simulink model "ProposedProblem1"  (R2013a)
settings: Solver=ode45  StartTime=0.0  StopTime=100  RelTol=1e-3
undefined symbols (not defined in the file): des, gcbh
settings Model: Creator=gabig  LastModifiedBy=gabig

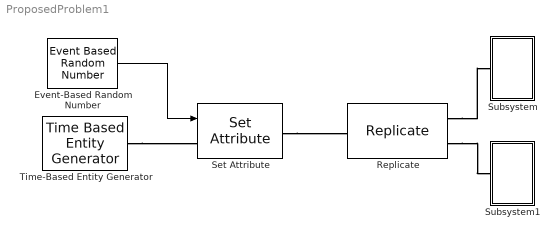
== system ProposedProblem1 ==
  Event-Based Random Number : EventBasedRandomNumber  Seed=14237
  Replicate : Replicate  NumberOutputPorts=2
  Set Attribute : SetAttribute  AttributeName=ServTime  AttributeFrom=Signal port  EvaluatedAttributeValue={ []}
  Subsystem : Subsystem
  Subsystem1 : Subsystem
  Time-Based Entity Generator : TimeBasedEntityGenerator  Distribution=Exponential  Mean=0.5
  wires:
  Event-Based Random Number/1 -> Set Attribute/1
  connections:
  Replicate/RConn2 -- Subsystem1/LConn1
  Time-Based Entity Generator/RConn1 -- Set Attribute/LConn1
  Replicate/RConn1 -- Subsystem/LConn1
  Set Attribute/RConn1 -- Replicate/LConn1

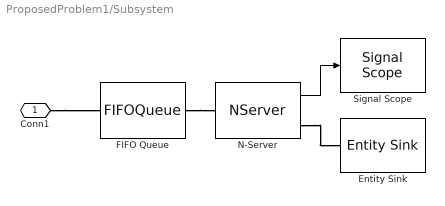
== system ProposedProblem1/Subsystem ==
  Entity Sink : EntitySink
  FIFO Queue : FIFOQueue
  N-Server : NServer  NumberOfServers=2  StatNumberDeparted=on
  Signal Scope : SignalScope  LoadFcn=des.scope.CallbackSupport('seLoadFcn',gcbh)  StartFcn=des.scope.CallbackSupport('seStartFcn',gcbh)  StopFcn=des.scope.CallbackSupport('seStopFcn',gcbh)  ShowCountPlotted=on
      settings: CopyFcn=des.scope.CallbackSupport('seCopyFcn',gcbh)  DeleteFcn=des.scope.CallbackSupport('seDeleteFcn',gcbh)  PreSaveFcn=des.scope.CallbackSupport('sePreSaveFcn',gcbh)  NameChangeFcn=des.scope.CallbackSupport('seNameChangeFcn',gcbh)  OpenFcn=des.scope.CallbackSupport('seOpenFcn',gcbh)
  Conn1 : PMIOPort  Port=1  Side=Left
  wires:
  N-Server/1 -> Signal Scope/1
  connections:
  Conn1/RConn1 -- FIFO Queue/LConn1
  N-Server/RConn1 -- Entity Sink/LConn1
  FIFO Queue/RConn1 -- N-Server/LConn1

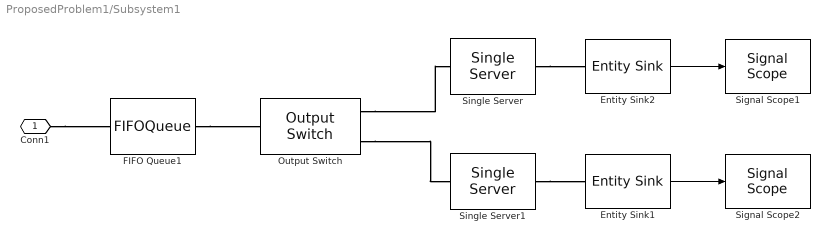
== system ProposedProblem1/Subsystem1 ==
  Entity Sink1 : EntitySink  StatNumberArrived=on
  Entity Sink2 : EntitySink  StatNumberArrived=on
  FIFO Queue1 : FIFOQueue
  Output Switch : OutputSwitch  NumberOutputPorts=2
  Signal Scope1 : SignalScope  LoadFcn=des.scope.CallbackSupport('seLoadFcn',gcbh)  StartFcn=des.scope.CallbackSupport('seStartFcn',gcbh)  StopFcn=des.scope.CallbackSupport('seStopFcn',gcbh)  ShowCountPlotted=on
      settings: CopyFcn=des.scope.CallbackSupport('seCopyFcn',gcbh)  DeleteFcn=des.scope.CallbackSupport('seDeleteFcn',gcbh)  PreSaveFcn=des.scope.CallbackSupport('sePreSaveFcn',gcbh)  NameChangeFcn=des.scope.CallbackSupport('seNameChangeFcn',gcbh)  OpenFcn=des.scope.CallbackSupport('seOpenFcn',gcbh)
  Signal Scope2 : SignalScope  LoadFcn=des.scope.CallbackSupport('seLoadFcn',gcbh)  StartFcn=des.scope.CallbackSupport('seStartFcn',gcbh)  StopFcn=des.scope.CallbackSupport('seStopFcn',gcbh)  ShowCountPlotted=on
      settings: CopyFcn=des.scope.CallbackSupport('seCopyFcn',gcbh)  DeleteFcn=des.scope.CallbackSupport('seDeleteFcn',gcbh)  PreSaveFcn=des.scope.CallbackSupport('sePreSaveFcn',gcbh)  NameChangeFcn=des.scope.CallbackSupport('seNameChangeFcn',gcbh)  OpenFcn=des.scope.CallbackSupport('seOpenFcn',gcbh)
  Single Server : SingleServer
  Single Server1 : SingleServer
  Conn1 : PMIOPort  Port=1  Side=Left
  wires:
  Entity Sink1/1 -> Signal Scope2/1
  Entity Sink2/1 -> Signal Scope1/1
  connections:
  Single Server/RConn1 -- Entity Sink2/LConn1
  Single Server1/RConn1 -- Entity Sink1/LConn1
  Conn1/RConn1 -- FIFO Queue1/LConn1
  FIFO Queue1/RConn1 -- Output Switch/LConn1
  Output Switch/RConn1 -- Single Server/LConn1
  Output Switch/RConn2 -- Single Server1/LConn1
